simulink model "statsim"  (R2022a)
settings: Solver=ode23  StartTime=0.00  StopTime=T  MaxStep=0.1  RelTol=1e-3
values from neighbouring files (symbols this model uses):
  a = (v([2:end 1],:)-v([end 1:end-1],:))./T./2    [elvio_resample.m]
  k = kp.*0    [stat_k.m]
  k_av = [1;2*v0;v0^2]*kp_av    [stat_k.m]
  kp = [ ... (first row only)    [stat_kp.m]
  kp_av = a(1)*m^2    [stat_kp.m]
  v = interp1(ct,cv,t)    [elvio_resample.m]
  v0 = mean(v)    [elvio_resample.m]
undefined symbols (not defined in the file or in its folder): alpha, c, m
settings Model: Creator=thomas  LastModifiedBy=elts2

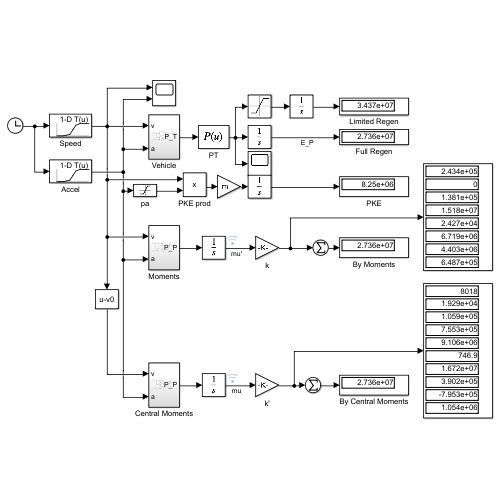
[thumbnail: Simulink's stored preview of the top-level diagram]
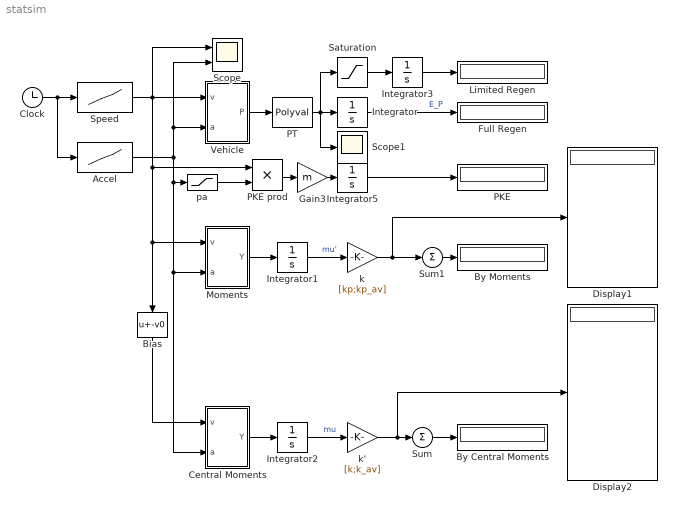
== system statsim ==
  Accel : Lookup_n-D  NumberOfTableDimensions=1  BreakpointsForDimension1=t  Table=a  ExtrapMethod=Clip  InternalRulePriority=Speed  RndMeth=Simplest
  Bias : Bias  Bias=-v0  SaturateOnIntegerOverflow=off
  By Central Moments : Display
  By Moments : Display
  Central Moments : Subsystem
  Clock : Clock
  Display1 : Display
  Display2 : Display
  Full Regen : Display
  Gain3 : Gain  Gain=m
  Integrator{,1..3,5} (5 alike) : Integrator
  Limited Regen : Display
  Moments : Subsystem
  PKE : Display
  PKE prod : Product
  PT : Polyval  Coefs=alpha
  Saturation : Saturate  UpperLimit=inf  LowerLimit=0
  Scope : Scope  NumInputPorts=2
  Scope1 : Scope
  Speed : Lookup_n-D  NumberOfTableDimensions=1  BreakpointsForDimension1=t  Table=v  ExtrapMethod=Clip  InternalRulePriority=Speed  RndMeth=Simplest
  Sum : Sum  Inputs=+
  Sum1 : Sum  Inputs=+
  Vehicle : Subsystem
  k : Gain  Gain=[kp;kp_av]
  k' : Gain  Gain=[k;k_av]
  pa : Saturate  UpperLimit=inf  LowerLimit=-0.2
  wires:
  Clock/1 -> Accel/1, Speed/1
  Speed/1 -> PKE prod/1, Bias/1, Moments/1(v), Vehicle/1(v), Scope/1
  PT/1 -> Scope1/1, Saturation/1, Integrator/1
  Integrator/1 -> Full Regen/1  "E_P"
  Integrator1/1 -> k/1  "mu'"
  Central Moments/1(Y) -> Integrator2/1
  Integrator2/1 -> k'/1  "mu"
  Moments/1(Y) -> Integrator1/1
  Vehicle/1(P) -> PT/1
  Sum/1 -> By Central Moments/1
  Bias/1 -> Central Moments/1(v)
  Accel/1 -> Vehicle/2(a), Scope/2, Central Moments/2(a), Moments/2(a), pa/1
  Saturation/1 -> Integrator3/1
  Integrator3/1 -> Limited Regen/1
  Sum1/1 -> By Moments/1
  Integrator5/1 -> PKE/1
  PKE prod/1 -> Gain3/1
  Gain3/1 -> Integrator5/1
  pa/1 -> PKE prod/2
  k/1 -> Display1/1, Sum1/1
  k'/1 -> Display2/1, Sum/1

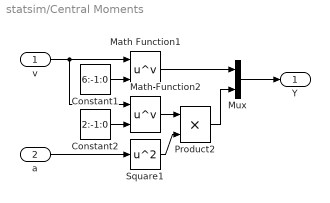
== system statsim/Central Moments ==
  v : Inport
  a : Inport  Port=2
  Constant1 : Constant  Value=6:-1:0
  Constant2 : Constant  Value=2:-1:0
  Math Function1 : Math  Operator=pow
  Math Function2 : Math  Operator=pow
  Mux : Mux  Inputs=2
  Product2 : Product
  Square1 : Math  Operator=square
  Y : Outport
  wires:
  Mux/1 -> Y/1
  Constant2/1 -> Math Function2/2
  Square1/1 -> Product2/2
  v/1 -> Math Function2/1, Math Function1/1
  Math Function2/1 -> Product2/1
  Math Function1/1 -> Mux/1
  Product2/1 -> Mux/2
  Constant1/1 -> Math Function1/2
  a/1 -> Square1/1

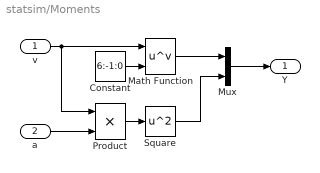
== system statsim/Moments ==
  v : Inport
  a : Inport  Port=2
  Constant : Constant  Value=6:-1:0
  Math Function : Math  Operator=pow
  Mux : Mux  Inputs=2
  Product : Product
  Square : Math  Operator=square
  Y : Outport
  wires:
  Mux/1 -> Y/1
  Constant/1 -> Math Function/2
  Product/1 -> Square/1
  Square/1 -> Mux/2
  Math Function/1 -> Mux/1
  v/1 -> Product/1, Math Function/1
  a/1 -> Product/2

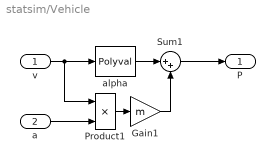
== system statsim/Vehicle ==
  v : Inport
  a : Inport  Port=2
  Gain1 : Gain  Gain=m
  Product1 : Product
  Sum1 : Sum  Inputs=|++
  alpha : Polyval  Coefs=[c 0]
  P : Outport
  wires:
  Product1/1 -> Gain1/1
  Gain1/1 -> Sum1/2
  alpha/1 -> Sum1/1
  v/1 -> Product1/1, alpha/1
  Sum1/1 -> P/1
  a/1 -> Product1/2
